simulink subsystem "DeserializeUINT32"  (R2019b)
settings: Solver=VariableStepAuto  StartTime=0.0  StopTime=10.0  RelTol=1e-3
undefined symbols (not defined in the file or in its folder): __PRM__SERIALIZED__DATA__, SubsystemReferenceBlock
settings Model: Creator=VM  LastModifiedBy=VM

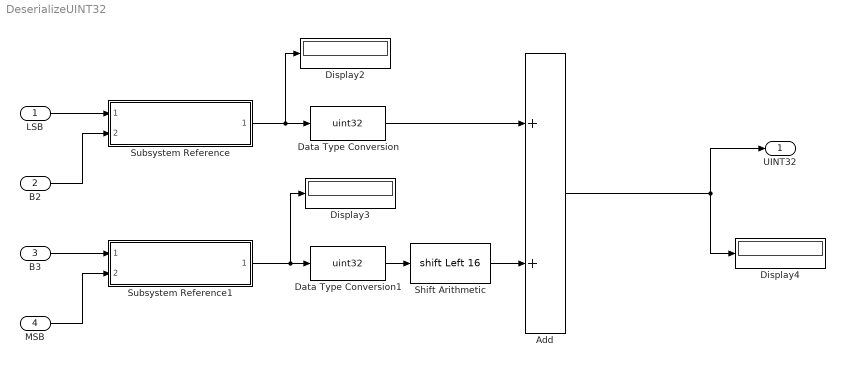
== system DeserializeUINT32 ==
  LSB : Inport  OutDataTypeStr=uint8
  B2 : Inport  Port=2  OutDataTypeStr=uint8
  B3 : Inport  Port=3  OutDataTypeStr=uint8
  MSB : Inport  Port=4  OutDataTypeStr=uint8
  Add : Sum
  Data Type Conversion : DataTypeConversion  OutDataTypeStr=uint32
  Data Type Conversion1 : DataTypeConversion  OutDataTypeStr=uint32
  Display2 : Display
  Display3 : Display
  Display4 : Display
  Shift Arithmetic : ArithShift  BitShiftNumber=16  BitShiftDirection=Left
  Subsystem Reference : Subsystem  BlockKeywords=__PRM__SERIALIZED__DATA__:SubsystemReferenceBlock  ReferencedSubsystem=DeserializeUINT16
  Subsystem Reference1 : Subsystem  BlockKeywords=__PRM__SERIALIZED__DATA__:SubsystemReferenceBlock  ReferencedSubsystem=DeserializeUINT16
  UINT32 : Outport  OutDataTypeStr=uint32  LockScale=on
  wires:
  MSB/1 -> Subsystem Reference1/2
  B3/1 -> Subsystem Reference1/1
  B2/1 -> Subsystem Reference/2
  LSB/1 -> Subsystem Reference/1
  Subsystem Reference/1 -> Display2/1, Data Type Conversion/1
  Subsystem Reference1/1 -> Display3/1, Data Type Conversion1/1
  Data Type Conversion1/1 -> Shift Arithmetic/1
  Add/1 -> Display4/1, UINT32/1
  Data Type Conversion/1 -> Add/1
  Shift Arithmetic/1 -> Add/2
